simulink model "sineIntegral"  (R2018a)
settings: Solver=ode45  StartTime=0.0  StopTime=50  RelTol=1e-3  EnableMultiTasking=on
settings Model: Creator=jrivitus  LastModifiedBy=bneiswan
settings DataIOCC: LimitDataPoints=on  SaveFormat=Array
settings OptimizationCC: ExpressionDepthLimit=2147483647  InitFltsAndDblsToZero=on  LifeSpan=inf
settings DebuggingCC: UnderspecifiedInitializationDetection=Classic  MergeDetectMultiDrivingBlocksExec=none  ParameterPrecisionLossMsg=none  FcnCallInpInsideContextMsg=warning  AllowSymbolicDim=off  StateNameClashWarn=warning  SFUnexpectedBacktrackingDiag=warning  SFNoUnconditionalDefaultTransitionDiag=warning  SFExecutionAtInitializationDiag=none
settings HardwareCC: ProdBitPerPointer=32  ProdBitPerSizeT=32  ProdBitPerPtrDiffT=32  ProdLargestAtomicFloat=None  ProdIntDivRoundTo=Undefined  ProdEndianess=Unspecified  ProdWordSize=32  ProdHWDeviceType=32-bit Generic
settings ModelReferenceCC: PropagateSignalLabelsOutOfModel=off
settings CodeAppCC: StateflowObjectComments=on
settings GRTTargetCC: TargetLangStandard=C89/C90 (ANSI)  GeneratePreprocessorConditionals=Disable all  CombineOutputUpdateFcns=off  GRTInterface=on
settings ConfigComp: CovMetricSettings=dw  CovHtmlReporting=on  CovSaveCumulativeToWorkspaceVar=on  CovSaveSingleToWorkspaceVar=on  CovExternalEMLEnable=off  CovSFcnEnable=off

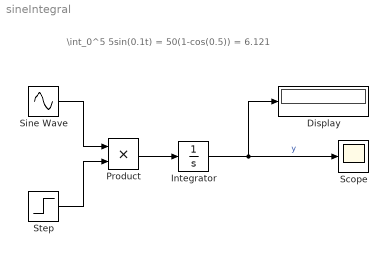
== system sineIntegral ==
  note: \int_0^5 5sin(0.1t) = 50(1-cos(0.5)) = 6.121
  Display : Display
  Integrator : Integrator
  Product : Product  RndMeth=Zero
  Scope : Scope
  Sine Wave : Sin  Amplitude=5  Frequency=0.1  SampleTime=0
      settings: AttributesFormatString=Amplitude: %<Amplitude>\nFrequency: %<Frequency>
  Step : Step  Time=5  Before=1  After=0  SampleTime=0
      settings: AttributesFormatString=Step time: %<Time>\nInitial value: %<Before>\nFinal value: %<After>
  wires:
  Integrator/1 -> Scope/1, Display/1  "y"
  Product/1 -> Integrator/1
  Sine Wave/1 -> Product/1
  Step/1 -> Product/2
